simulink model "EngineWcControl"  (Simulink 7.7)
settings: Solver=ode45  StartTime=0.0  StopTime=10.0  RelTol=1e-3
values from neighbouring files (symbols this model uses):
  Ki = 0.0723    [initEngineWcControl.m]
  Kp = 0.0614    [initEngineWcControl.m]
  pi_user = 3.141592654    [initEngineWcControl.m]
undefined symbols (not defined in the file or in its folder): DiscIntNeverNeededParam
settings Model: Creator=sundu  LastModifiedBy=sundu

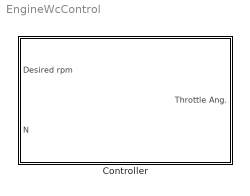
== system EngineWcControl ==
  Controller : Subsystem  TreatAsAtomicUnit=on

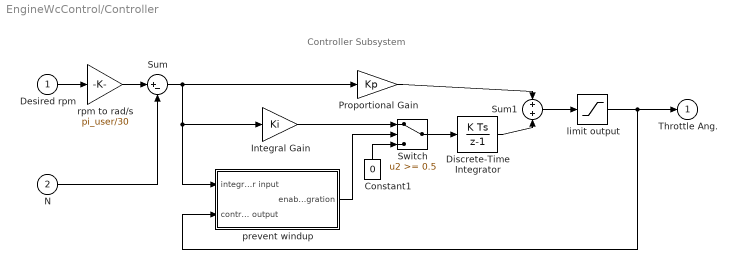
== system EngineWcControl/Controller ==
  note: Controller Subsystem
  Desired rpm : Inport
  N : Inport  Port=2
  Constant1 : Constant  Value=0
  Discrete-Time Integrator : DiscreteIntegrator  InitialCondition=8.973  SampleTime=-1  ICPrevOutput=DiscIntNeverNeededParam  ICPrevScaledInput=DiscIntNeverNeededParam
  Integral Gain : Gain  Gain=Ki  SaturateOnIntegerOverflow=on  OutDataTypeStr=Inherit: Same as input  ParamDataTypeStr=Inherit: Same as input
  Proportional Gain : Gain  Gain=Kp  SaturateOnIntegerOverflow=on  OutDataTypeStr=Inherit: Same as input  ParamDataTypeStr=Inherit: Same as input
  Sum : Sum  Inputs=|+-  SaturateOnIntegerOverflow=on  InputSameDT=on  OutDataTypeStr=Inherit: Same as first input
  Sum1 : Sum  SaturateOnIntegerOverflow=on  InputSameDT=on  OutDataTypeStr=Inherit: Same as first input
  Switch : Switch  Threshold=0.5  SaturateOnIntegerOverflow=on  InputSameDT=on
  limit output : Saturate  UpperLimit=70  LowerLimit=0
  prevent windup : Subsystem
  rpm to rad/s : Gain  Gain=pi_user/30  SaturateOnIntegerOverflow=on  OutDataTypeStr=Inherit: Same as input  ParamDataTypeStr=Inherit: Same as input
  Throttle Ang. : Outport  InitialOutput=8.973
  wires:
  rpm to rad/s/1 -> Sum/1
  Discrete-Time Integrator/1 -> Sum1/2
  limit output/1 -> prevent windup/2(controller output), Throttle Ang./1
  prevent windup/1(enable integration) -> Switch/2
  Sum1/1 -> limit output/1
  Switch/1 -> Discrete-Time Integrator/1
  Proportional Gain/1 -> Sum1/1
  Constant1/1 -> Switch/3
  Integral Gain/1 -> Switch/1
  Sum/1 -> prevent windup/1(integrator input), Integral Gain/1, Proportional Gain/1
  N/1 -> Sum/2
  Desired rpm/1 -> rpm to rad/s/1

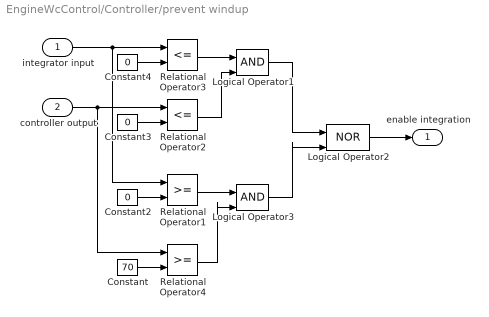
== system EngineWcControl/Controller/prevent windup ==
  integrator input : Inport
  controller output : Inport  Port=2
  Constant : Constant  Value=70
  Constant2 : Constant  Value=0
  Constant3 : Constant  Value=0
  Constant4 : Constant  Value=0
  Logical Operator1 : Logic  IconShape=distinctive
  Logical Operator2 : Logic  Operator=NOR  IconShape=distinctive
  Logical Operator3 : Logic  IconShape=distinctive
  Relational Operator1 : RelationalOperator  InputSameDT=on
  Relational Operator2 : RelationalOperator  Operator=<=  InputSameDT=on
  Relational Operator3 : RelationalOperator  Operator=<=  InputSameDT=on
  Relational Operator4 : RelationalOperator  InputSameDT=on
  enable integration : Outport  InitialOutput=0
  wires:
  Logical Operator2/1 -> enable integration/1
  Logical Operator3/1 -> Logical Operator2/2
  Logical Operator1/1 -> Logical Operator2/1
  Relational Operator4/1 -> Logical Operator3/2
  Relational Operator1/1 -> Logical Operator3/1
  Constant/1 -> Relational Operator4/2
  Constant2/1 -> Relational Operator1/2
  controller output/1 -> Relational Operator4/1, Relational Operator2/1
  integrator input/1 -> Relational Operator3/1, Relational Operator1/1
  Relational Operator2/1 -> Logical Operator1/2
  Relational Operator3/1 -> Logical Operator1/1
  Constant4/1 -> Relational Operator3/2
  Constant3/1 -> Relational Operator2/2
